simulink model "missile_project"  (R2024b)
settings: Solver=VariableStepAuto  StartTime=0.0  StopTime=80  RelTol=1e-3
undefined symbols (not defined in the file): A, B, C, D, dT1, dT2, Earth, ELEV_INIT, ELEV_TARGET, K, L, LAT_INIT, LAT_OBS, LAT_TARGET, LON_INIT, LON_OBS, LON_TARGET, Vel, WGS84
libraries: simulink x3, slpidlib x1, aerolibtransform2 x1, aerolibanimutils x1
settings Model: Creator=mglab  LastModifiedBy=mglab

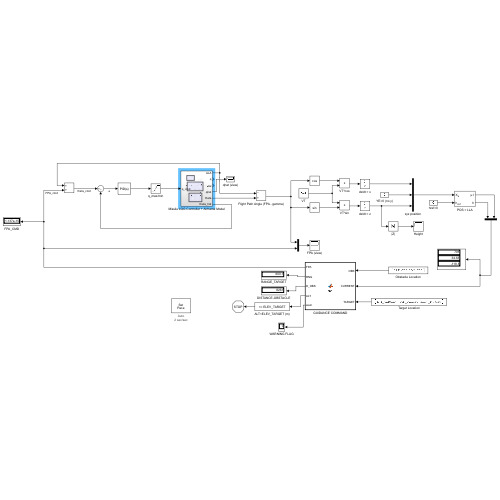
[thumbnail: Simulink's stored preview of the top-level diagram]
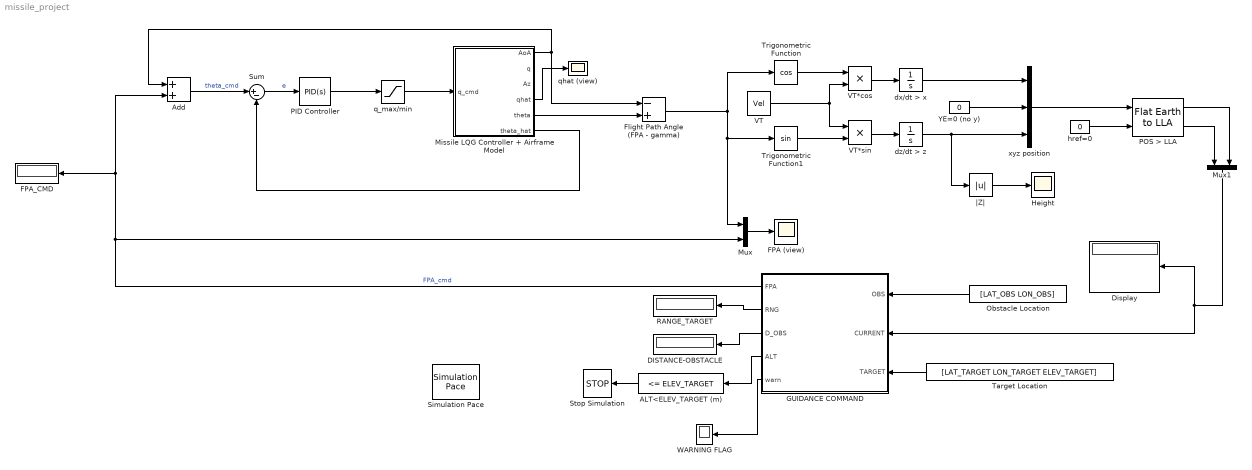
== system missile_project ==
  ALT<ELEV_TARGET (m) : simulink/Logic and Bit Operations/Compare To Constant  relop=<=  const=ELEV_TARGET  OutDataTypeStr=boolean
  Add : Sum
  DISTANCE-OBSTACLE : Display
  Display : Display
  FPA (view) : Scope
  FPA_CMD : Display
  Flight Path Angle (FPA - gamma) : Sum  Inputs=-+
  GUIDANCE COMMAND : MATLAB Function  TreatAsAtomicUnit=on
  Height : Scope
  Missile LQG Controller + Airframe Model : Subsystem
  Mux : Mux  Inputs=2
  Mux1 : Mux  Inputs=2
  Obstacle Location : Constant  Value=[LAT_OBS LON_OBS]
  PID Controller : slpidlib/PID Controller  Controller=PID  Form=Parallel  TimeDomain=Continuous-time  UseExternalTs=off  SampleTime=-1  IntegratorMethod=Forward Euler  FilterMethod=Forward Euler  ControllerParametersSource=internal  P=-1  I=0  UseKiTs=off  D=0  UseExternalDerivativeSource=off  N=100  UseFilter=on  TunerSelectOption=Transfer Function Based (PID Tuner App)  InitialConditionSource=internal  InitialConditionForIntegrator=0  InitialConditionForFilter=0  DifferentiatorICPrevScaledInput=0  ExternalReset=none  TrackingMode=off  Kt=1  LimitOutput=off  SatLimitsSource=internal  UpperSaturationLimit=inf  LowerSaturationLimit=-inf  LinearizeAsGain=on  AntiWindupMode=none  Kb=1  LimitIntegrator=off  UpperIntegratorSaturationLimit=inf  LowerIntegratorSaturationLimit=-inf  POutMin=[]  POutMax=[]  IOutMin=[]  IOutMax=[]  DOutMin=[]  DOutMax=[]  NOutMin=[]  NOutMax=[]  SumOutMin=[]  SumOutMax=[]  SaturationOutMin=[]  SaturationOutMax=[]  PParamMin=[]  PParamMax=[]  IParamMin=[]  IParamMax=[]  DParamMin=[]  DParamMax=[]  NParamMin=[]  NParamMax=[]  KbParamMin=[]  KbParamMax=[]  KtParamMin=[]  KtParamMax=[]  KbOutMin=[]  KbOutMax=[]  KtOutMin=[]  KtOutMax=[]  IntegratorOutMin=[]  IntegratorOutMax=[]  FilterOutMin=[]  FilterOutMax=[]  SumI1OutMin=[]  SumI1OutMax=[]  SumI2OutMin=[]  SumI2OutMax=[]  SumI3OutMin=[]  SumI3OutMax=[]  SumI4OutMin=[]  SumI4OutMax=[]  SumDOutMin=[]  SumDOutMax=[]  DifferentiatorOutMin=[]  DifferentiatorOutMax=[]  FilterDiffOutCoefMin=[]  FilterDiffOutCoefMax=[]  ReciprocalOutMin=[]  ReciprocalOutMax=[]  SumDenOutMin=[]  SumDenOutMax=[]  SumNumOutMin=[]  SumNumOutMax=[]  DivideOutMin=[]  DivideOutMax=[]  UdiffTsProdOutMin=[]  UdiffTsProdOutMax=[]  NTsProdOutMin=[]  NTsProdOutMax=[]  UintegralTsProdOutMin=[]  UintegralTsProdOutMax=[]  UngainTsProdOutMin=[]  UngainTsProdOutMax=[]  ClampingZeroOutDataTypeStr=Inherit: Inherit via back propagation  ClampingZeroOutMin=[]  ClampingZeroOutMax=[]  FilterDenConstantOutDataTypeStr=Inherit: Inherit via back propagation  FilterDenConstantOutMin=[]  FilterDenConstantOutMax=[]  PCopyOutDataTypeStr=Inherit: Inherit via back propagation  PCopyOutMin=[]  PCopyOutMax=[]  NCopyOutDataTypeStr=Inherit: Inherit via back propagation  NCopyOutMin=[]  NCopyOutMax=[]  IntegratorContinuousStateAttributes=''  IntegratorStateMustResolveToSignalObject=off  IntegratorRTWStateStorageClass=Auto  FilterContinuousStateAttributes=''  FilterStateMustResolveToSignalObject=off  FilterRTWStateStorageClass=Auto  ParallelPVariant=InternalParameters  IdealPVariant=Disabled  IVariant=InternalParameters  DVariant=InternalParameters  IntegratorVariant=Continuous  SatVariant=Disabled  AWVariant=Passthrough  PCopyVariant=Disabled  TRVariant=Disabled  FdbkBlocksVariant=Forward  IdealPFdbkVariant=Disabled  SatFdbkVariant=Disabled  DerivativeFilterVariant=ContFilter  NVariant=InternalParameters  NCopyVariant=Disabled  FilterICVariant=InternalICsFilter  IntegratorICVariant=InternalICs  ExternalResetVariant=Disabled  TRSumVariant=Passthrough  SumFdbkVariant=Disabled  SumVariant=Sum_PID  TsampFilterVariant=InternalTs  TsampNgainVariant=Passthrough  TsampIntegralVariant=Disabled_SignalSpec  ExternalSaturationOutDataTypeStr=Inherit: Same as second input  DerivativeSourceVariant=ErrorSignal  PreIntVariant=InternalPreInt
  POS > LLA : aerolibtransform2/Flat Earth to LLA  units=Metric (MKS)  ptype=Earth (WGS84)  F=1/298.257223563  R=6378137  refPosPort=off  LL0=[LAT_INIT LON_INIT]  psi=yaw_init
  RANGE_TARGET : Display
  Simulation Pace : aerolibanimutils/Simulation Pace  SimulationPace=2  SleepMode=Auto  OutputPaceError=off  SampleTime=1/30
  Stop Simulation : Stop
  Sum : Sum  Inputs=|+-
  Target Location : Constant  Value=[LAT_TARGET LON_TARGET ELEV_TARGET]
  Trigonometric Function : Trigonometry  Operator=cos
  Trigonometric Function1 : Trigonometry
  VT : Constant  Value=Vel
  VT*cos : Product
  VT*sin : Product
  WARNING FLAG : Display
  YE=0 (no y) : Constant  Value=0
  dx/dt > x : Integrator
  dz/dt > z : Integrator  InitialCondition=-ELEV_INIT
  href=0 : Constant  Value=0
  q_max/min : Saturate
  qhat (view) : Scope
  xyz position : Mux  Inputs=3
  |Z| : Abs  SaturateOnIntegerOverflow=off
  wires:
  PID Controller/1 -> q_max/min/1
  q_max/min/1 -> Missile LQG Controller + Airframe Model/1(q_cmd)
  Sum/1 -> PID Controller/1  "e"
  Missile LQG Controller + Airframe Model/6(theta_hat) -> Sum/2
  Add/1 -> Sum/1  "theta_cmd"
  Missile LQG Controller + Airframe Model/1(AoA) -> Flight Path Angle (FPA - gamma)/1, Add/1
  Missile LQG Controller + Airframe Model/5(theta) -> Flight Path Angle (FPA - gamma)/2
  GUIDANCE COMMAND/1(FPA) -> Add/2, FPA_CMD/1, Mux/2  "FPA_cmd"
  Flight Path Angle (FPA - gamma)/1 -> Trigonometric Function/1, Trigonometric Function1/1, Mux/1
  Mux/1 -> FPA (view)/1
  Trigonometric Function1/1 -> VT*sin/2
  Trigonometric Function/1 -> VT*cos/1
  VT/1 -> VT*cos/2, VT*sin/1
  VT*sin/1 -> dz/dt > z/1
  VT*cos/1 -> dx/dt > x/1
  dx/dt > x/1 -> xyz position/1
  YE=0 (no y)/1 -> xyz position/2
  dz/dt > z/1 -> |Z|/1, xyz position/3
  |Z|/1 -> Height/1
  xyz position/1 -> POS > LLA/1
  href=0/1 -> POS > LLA/2
  POS > LLA/2 -> Mux1/1
  POS > LLA/1 -> Mux1/2
  Obstacle Location/1 -> GUIDANCE COMMAND/1(OBS)
  Target Location/1 -> GUIDANCE COMMAND/3(TARGET)
  Mux1/1 -> Display/1, GUIDANCE COMMAND/2(CURRENT)
  GUIDANCE COMMAND/2(RNG) -> RANGE_TARGET/1
  GUIDANCE COMMAND/3(D_OBS) -> DISTANCE-OBSTACLE/1
  GUIDANCE COMMAND/5(warn) -> WARNING FLAG/1
  GUIDANCE COMMAND/4(ALT) -> ALT<ELEV_TARGET (m)/1
  ALT<ELEV_TARGET (m)/1 -> Stop Simulation/1
  Missile LQG Controller + Airframe Model/4(qhat) -> qhat (view)/1

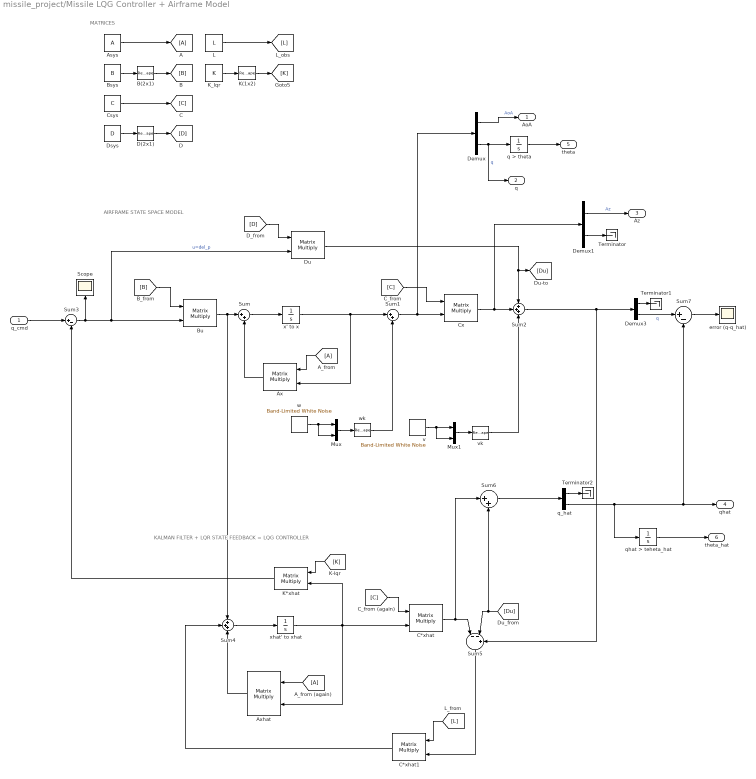
== system missile_project/Missile LQG Controller + Airframe Model ==
  note: KALMAN FILTER + LQR STATE FEEDBACK = LQG CONTROLLER
  note: AIRFRAME STATE SPACE MODEL
  note: MATRICES
  q_cmd : Inport
  A : Goto
  A_from : From
  A_from (again) : From
  Asys : Constant  Value=A
  Ax : Product  Multiplication=Matrix(*)
  Axhat : Product  Multiplication=Matrix(*)
  B(2x1) : Reshape  OutputDimensionality=Customize  OutputDimensions=[2,1]
  Bsys : Constant  Value=B
  Bu : Product  Multiplication=Matrix(*)
  C*xhat : Product  Multiplication=Matrix(*)
  C*xhat1 : Product  Multiplication=Matrix(*)
  Csys : Constant  Value=C
  Cx : Product  Multiplication=Matrix(*)
  D(2x1) : Reshape  OutputDimensionality=Customize  OutputDimensions=[2,1]
  Demux : Demux  Outputs=2
  Demux1 : Demux  Outputs=2
  Demux3 : Demux  Outputs=2
  Dsys : Constant  Value=D
  Du : Product  Multiplication=Matrix(*)
  K(1x2) : Reshape  OutputDimensionality=Customize  OutputDimensions=[1,2]
  K*xhat : Product  Multiplication=Matrix(*)
  K_lqr : Constant  Value=K
  L : Constant  Value=L
  Mux : Mux  Inputs=2
  Mux1 : Mux  Inputs=2
  Scope : Scope
  Sum : Sum  Inputs=|++
  Sum1 : Sum  Inputs=|++
  Sum2 : Sum  Inputs=+++
  Sum3 : Sum  Inputs=|+-
  Sum4 : Sum  Inputs=+++
  Sum5 : Sum  Inputs=|--+
  Sum6 : Sum  Inputs=|++
  Sum7 : Sum  Inputs=|+-
  Terminator : Terminator
  Terminator1 : Terminator
  Terminator2 : Terminator
  error (q-q_hat) : Scope
  q > theta : Integrator
  q_hat : Demux  Outputs=2
  qhat > teheta_hat : Integrator
  v : simulink/Sources/Band-Limited White Noise  Cov=[0.00001]  Ts=dT2  seed=[23341]
  vk : Reshape  OutputDimensionality=Customize  OutputDimensions=[2,1]
  w : simulink/Sources/Band-Limited White Noise  Cov=[0.00000001]  Ts=dT1  seed=[23341]
  wk : Reshape  OutputDimensionality=Customize  OutputDimensions=[2,1]
  x' to x : Integrator
  xhat' to xhat : Integrator
  AoA : Outport
  q : Outport  Port=2
  Az : Outport  Port=3
  qhat : Outport  Port=4
  theta : Outport  Port=5
  theta_hat : Outport  Port=6
  wires:
  K*xhat/1 -> Sum3/2
  Cx/1 -> Demux1/1, Sum2/2
  Bsys/1 -> B(2x1)/1
  Sum3/1 -> Du/2, Bu/2, Scope/1  "u=del_p"
  x' to x/1 -> Ax/2, Sum1/1
  q_hat/2 -> qhat > teheta_hat/1, qhat/1, Sum7/2
  K_lqr/1 -> K(1x2)/1
  w/1 -> Mux/2, Mux/1
  Sum7/1 -> error (q-q_hat)/1
  [C] -> C*xhat/1
  Demux/2 -> q/1, q > theta/1  "q"
  [Du] -> Sum6/2, Sum5/2
  Asys/1 -> A/1
  wk/1 -> Sum1/2
  v/1 -> Mux1/2, Mux1/1
  Demux1/2 -> Terminator/1
  Sum4/1 -> xhat' to xhat/1
  Demux/1 -> AoA/1  "AoA"
  B(2x1)/1 -> [B]
  Sum/1 -> x' to x/1
  Bu/1 -> Sum/1, Sum4/1
  Sum1/1 -> Demux/1, Cx/2
  Sum2/1 -> Sum5/3, Demux3/1
  Du/1 -> [Du], Sum2/1
  [B] -> Bu/1
  Mux/1 -> wk/1
  [K] -> K*xhat/1
  A_from (again)/1 -> Axhat/1
  Ax/1 -> Sum/2
  Demux3/1 -> Terminator1/1
  [C] -> Cx/1
  Sum6/1 -> q_hat/1
  C*xhat/1 -> Sum6/1, Sum5/1
  A_from/1 -> Ax/1
  [L] -> C*xhat1/1
  L/1 -> [L]
  Demux3/2 -> Sum7/1  "q"
  Sum5/1 -> C*xhat1/2
  vk/1 -> Sum2/3
  [D] -> Du/1
  Axhat/1 -> Sum4/3
  Csys/1 -> [C]
  xhat' to xhat/1 -> K*xhat/2, C*xhat/2, Axhat/2
  Mux1/1 -> vk/1
  D(2x1)/1 -> [D]
  C*xhat1/1 -> Sum4/2
  q > theta/1 -> theta/1
  Demux1/1 -> Az/1  "Az"
  K(1x2)/1 -> [K]
  qhat > teheta_hat/1 -> theta_hat/1
  q_cmd/1 -> Sum3/1
  Dsys/1 -> D(2x1)/1
  q_hat/1 -> Terminator2/1

== matlab function missile_project/GUIDANCE COMMAND ==
  data: OBS input; FPA output; CURRENT input; TARGET input; RNG output; D_OBS output; ALT output; warn output
function [FPA,RNG,D_OBS,ALT,warn] = fcn(OBS, CURRENT, TARGET)

R = 6371e3;
d2r = pi/180;

%OBSTACLE LOCATION
LAT_OBS = OBS(1);
LON_OBS = OBS(2);

%OBSTACLE THRESHHOLD (ZONE)
thres = 2000; %2km

%TARGET LOCATION
LAT_TARGET = TARGET(1);
LON_TARGET = TARGET(2); 
ELEV_TARGET = TARGET(3); %m-MSL

%CURRENT LOCATION
ELEV_CUR = CURRENT(1);
LAT_CUR = CURRENT(2);
LON_CUR = CURRENT(3);

%% distance to target
l1 = LAT_CUR*d2r; 
u1 = LON_CUR*d2r; 
l2 = LAT_TARGET*d2r; 
u2 = LON_TARGET*d2r;
dh = abs(ELEV_TARGET-ELEV_CUR);

dl = l2-l1;
du = u2-u1;

a = sin(dl/2)^2 + cos(l1)*cos(l2)*sin(du/2)^2;
c = 2*atan2(sqrt(a), sqrt(1-a));
d = R*c; %horizontal distance (in m)

%% distance from the obstacle
l3 = LAT_OBS*d2r;
u3 = LON_OBS*d2r;

dl = l3-l1;
du = u3-u1;

a = sin(dl/2)^2 + cos(l1)*cos(l3)*sin(du/2)^2;
c = 2*atan2(sqrt(a), sqrt(1-a));
d_obs = R*c; %horizontal distance (in m)

%% current range (from target) - range > distance
range = sqrt(d^2+dh^2);

%% calculate commanded flight path setpoint based on d_obs, range
if abs(d_obs)>=thres
    w=0;  % flight path angle
    FPA_CMD = atan(dh/d);
else
    % when in the obstacle zone, trigger warning
    w = 1;
    FPA_CMD = 0;
end

%% output variables
FPA = FPA_CMD;
RNG = range;
D_OBS = d_obs;
warn = w;
ALT = ELEV_CUR;
